simulink model "lab1_extended_estimator"  (R2024b)
settings: Solver=ode45  StartTime=0.0  StopTime=sIn.simulation_time
values from neighbouring files (symbols this model uses):
  Ae = [ref_SS.A_r zeros(3,2); plant_SS.B*ref_SS.C_r plant_SS.A]    [lab1_startup_extended_estimator.m]
  Be = [zeros(3,1); plant_SS.B]    [lab1_startup_extended_estimator.m]
  Ce = [zeros(1,3) plant_SS.C]    [lab1_startup_extended_estimator.m]
undefined symbols (not defined in the file or in its folder): degs2rpm, drv, feedback, filt, gbox, mld, mot, rads2rpm, ref_SS, rpm2rads, sens, sIn, specs
libraries: simulink_extras x2
settings Model: Creator=bmm1  LastModifiedBy=Nihal
settings SolverCC: ZeroCrossAlgorithm=Adaptive
settings DebuggingCC: IgnoredZcDiagnostic=none
settings RTWCC: GPUComputeCapability=3.5

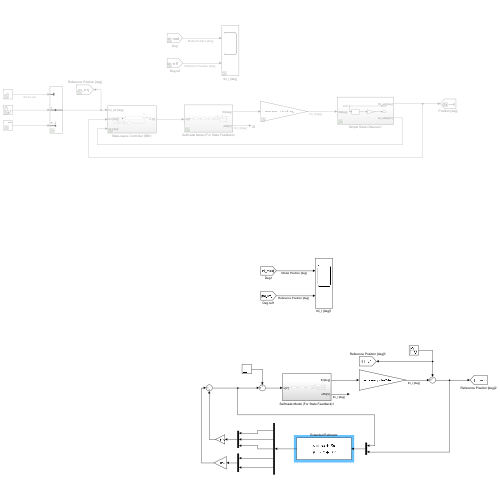
[thumbnail: Simulink's stored preview of the top-level diagram]
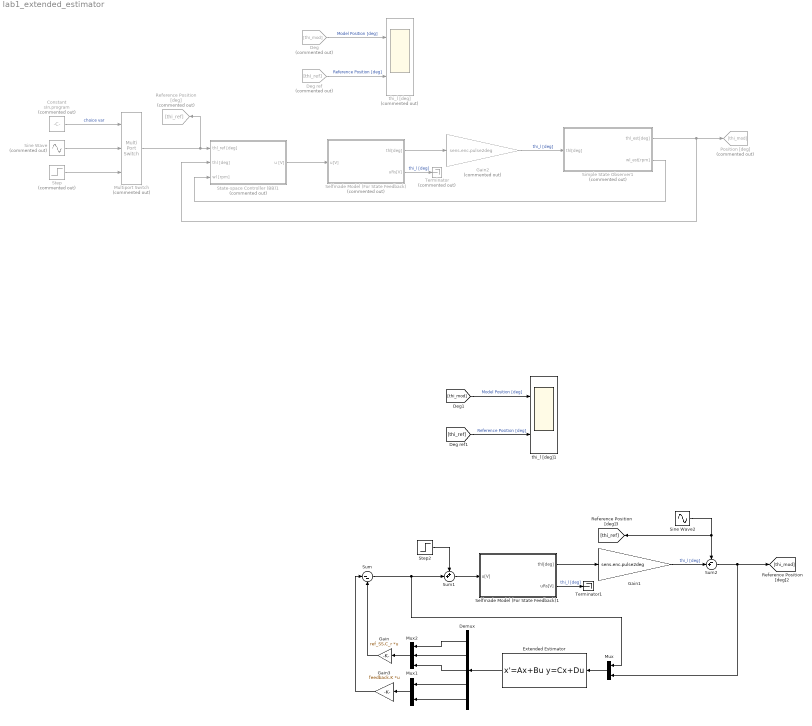
== system lab1_extended_estimator ==
  Constant : Constant  Commented=on  Value=sIn.program
  Deg : From  Commented=on  GotoTag=thi_mod
  Deg ref : From  Commented=on  GotoTag=thi_ref
  Demux : Demux  Outputs=5
  Extended Estimator : StateSpace  A=Ae - feedback.L*Ce  B=[Be, feedback.L]  C=eye(5,5)  D=zeros(5,2)  InitialCondition=0
  Gain : Gain  Gain=ref_SS.C_r  Multiplication=Matrix(K*u)
  Gain1 : Gain  Gain=sens.enc.pulse2deg
  Gain2 : Gain  Commented=on  Gain=sens.enc.pulse2deg
  Gain3 : Gain  Gain=feedback.K  Multiplication=Matrix(K*u)
  Multiport Switch : MultiPortSwitch  Commented=on  Inputs=2  SaturateOnIntegerOverflow=off  InputSameDT=off
  Mux : Mux  Inputs=2
  Mux1 : Mux  Inputs=2
  Mux2 : Mux  Inputs=3
  Position [deg] : Goto  Commented=on  GotoTag=thi_mod
  Reference Position [deg] : Goto  Commented=on  GotoTag=thi_ref
  Selfmade Model (For State Feedback) : Subsystem  Commented=on
  Selfmade Model (For State Feedback)1 : Subsystem
  Simple State Observer1 : Subsystem  Commented=on
  Sine Wave : Sin  Commented=on  Amplitude=specs.Amp  Frequency=specs.Freq  SampleTime=0
  Sine Wave2 : Sin  Amplitude=specs.Amp  Frequency=specs.Freq  SampleTime=0
  State-space Controller (BB)1 : Subsystem  Commented=on
  Step : Step  Commented=on  After=40  SampleTime=0
  Step2 : Step  After=40  SampleTime=0
  Sum : Sum  Inputs=|--
  Sum1 : Sum  Inputs=++|
  Sum2 : Sum  Inputs=-+|
  Terminator : Terminator  Commented=on
  Terminator1 : Terminator
  thi_l [deg] : Scope  Commented=on  NumInputPorts=2
  thi_l [deg]1 : Scope  NumInputPorts=2
  wires:
  Selfmade Model (For State Feedback)/1(thl[deg]) -> Gain2/1
  Deg/1 -> thi_l [deg]/1  "Model Position [deg]"
  Deg ref/1 -> thi_l [deg]/2  "Reference Position [deg]"
  State-space Controller (BB)1/1(u [V]) -> Selfmade Model (For State Feedback)/1(u[V])
  Selfmade Model (For State Feedback)/2(uRs[V]) -> Terminator/1  "thi_l [deg]"
  Gain2/1 -> Simple State Observer1/1(thl[deg])  "thi_l [deg]"
  Simple State Observer1/1(thl_est[deg]) -> Position [deg]/1, State-space Controller (BB)1/2(thl [deg])
  Simple State Observer1/2(wl_est[rpm]) -> State-space Controller (BB)1/3(wl [rpm])
  Sine Wave/1 -> Multiport Switch/2
  Multiport Switch/1 -> Reference Position [deg]/1, State-space Controller (BB)1/1(thl_ref [deg])
  Step/1 -> Multiport Switch/3
  Constant/1 -> Multiport Switch/1  "choice var"
  Selfmade Model (For State Feedback)1/2(uRs[V]) -> Terminator1/1  "thi_l [deg]"
  Sum/1 -> Sum1/2, Mux/1
  [thi_ref] -> thi_l [deg]1/2  "Reference Position [deg]"
  Selfmade Model (For State Feedback)1/1(thl[deg]) -> Gain1/1
  [thi_mod] -> thi_l [deg]1/1  "Model Position [deg]"
  Mux/1 -> Extended Estimator/1
  Extended Estimator/1 -> Demux/1
  Mux1/1 -> Gain3/1
  Demux/4 -> Mux1/1
  Demux/5 -> Mux1/2
  Demux/1 -> Mux2/1
  Demux/2 -> Mux2/2
  Demux/3 -> Mux2/3
  Mux2/1 -> Gain/1
  Gain/1 -> Sum/2
  Gain3/1 -> Sum/1
  Sum1/1 -> Selfmade Model (For State Feedback)1/1(u[V])
  Step2/1 -> Sum1/1
  Gain1/1 -> Sum2/2  "thi_l [deg]"
  Sine Wave2/1 -> Sum2/1, [thi_ref]
  Sum2/1 -> Mux/2, [thi_mod]

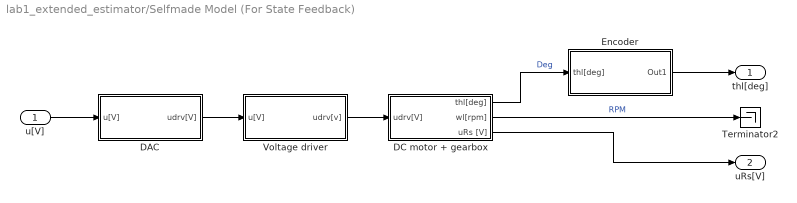
== system lab1_extended_estimator/Selfmade Model (For State Feedback) ==
  u[V] : Inport
  DAC : Subsystem
  DC motor + gearbox : Subsystem
  Encoder : Subsystem
  Terminator2 : Terminator
  Voltage driver : Subsystem
  thl[deg] : Outport
  uRs[V] : Outport  Port=2
  wires:
  DC motor + gearbox/1(thl[deg]) -> Encoder/1(thl[deg])  "Deg"
  u[V]/1 -> DAC/1(u[V])
  DC motor + gearbox/2(wl[rpm]) -> Terminator2/1  "RPM"
  DAC/1(udrv[V]) -> Voltage driver/1(u[V])
  Voltage driver/1(udrv[v]) -> DC motor + gearbox/1(udrv[V])
  Encoder/1(Out1) -> thl[deg]/1
  DC motor + gearbox/3(uRs [V]) -> uRs[V]/1

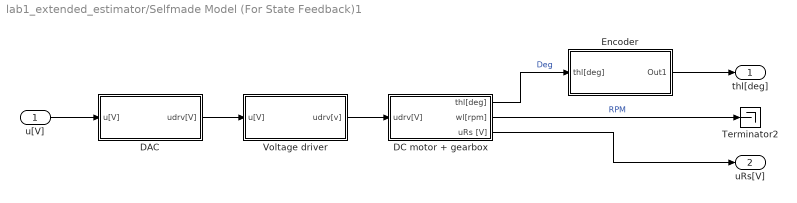
== system lab1_extended_estimator/Selfmade Model (For State Feedback)1 ==
  u[V] : Inport
  DAC : Subsystem
  DC motor + gearbox : Subsystem
  Encoder : Subsystem
  Terminator2 : Terminator
  Voltage driver : Subsystem
  thl[deg] : Outport
  uRs[V] : Outport  Port=2
  wires:
  DC motor + gearbox/1(thl[deg]) -> Encoder/1(thl[deg])  "Deg"
  u[V]/1 -> DAC/1(u[V])
  DC motor + gearbox/2(wl[rpm]) -> Terminator2/1  "RPM"
  DAC/1(udrv[V]) -> Voltage driver/1(u[V])
  Voltage driver/1(udrv[v]) -> DC motor + gearbox/1(udrv[V])
  Encoder/1(Out1) -> thl[deg]/1
  DC motor + gearbox/3(uRs [V]) -> uRs[V]/1

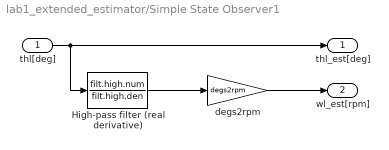
== system lab1_extended_estimator/Simple State Observer1 ==
  thl[deg] : Inport
  High-pass filter (real derivative) : TransferFcn  Numerator=filt.high.num  Denominator=filt.high.den
  degs2rpm : Gain  Gain=degs2rpm
  thl_est[deg] : Outport
  wl_est[rpm] : Outport  Port=2
  wires:
  thl[deg]/1 -> High-pass filter (real derivative)/1, thl_est[deg]/1
  High-pass filter (real derivative)/1 -> degs2rpm/1
  degs2rpm/1 -> wl_est[rpm]/1

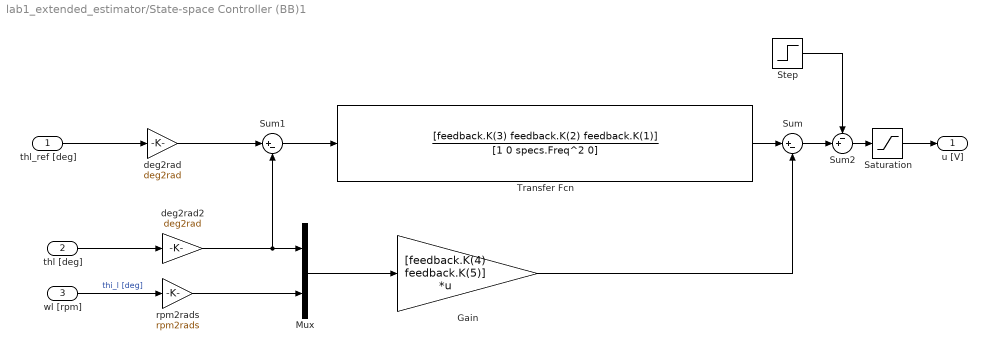
== system lab1_extended_estimator/State-space Controller (BB)1 ==
  thl_ref [deg] : Inport
  thl [deg] : Inport  Port=2
  wl [rpm] : Inport  Port=3
  Gain : Gain  Gain=[feedback.K(4) feedback.K(5)]  Multiplication=Matrix(K*u)
  Mux : Mux  Inputs=2
  Saturation : Saturate  UpperLimit=10  LowerLimit=-10
  Step : Step  After=40  SampleTime=0
  Sum : Sum  Inputs=|+-
  Sum1 : Sum  Inputs=|+-
  Sum2 : Sum  Inputs=-+|
  Transfer Fcn : TransferFcn  Numerator=[feedback.K(3) feedback.K(2) feedback.K(1)]  Denominator=[1 0 specs.Freq^2 0]
  deg2rad : Gain  Gain=deg2rad
  deg2rad2 : Gain  Gain=deg2rad
  rpm2rads : Gain  Gain=rpm2rads
  u [V] : Outport
  wires:
  thl_ref [deg]/1 -> deg2rad/1
  Transfer Fcn/1 -> Sum/1
  Saturation/1 -> u [V]/1
  thl [deg]/1 -> deg2rad2/1
  deg2rad2/1 -> Mux/1, Sum1/2
  deg2rad/1 -> Sum1/1
  Mux/1 -> Gain/1
  rpm2rads/1 -> Mux/2
  Gain/1 -> Sum/2
  Sum1/1 -> Transfer Fcn/1
  wl [rpm]/1 -> rpm2rads/1  "thi_l [deg]"
  Sum2/1 -> Saturation/1
  Sum/1 -> Sum2/2
  Step/1 -> Sum2/1

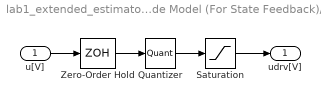
== system lab1_extended_estimator/Selfmade Model (For State Feedback)/DAC ==
  u[V] : Inport
  Quantizer : Quantizer  QuantizationInterval=daq.dac.q
  Saturation : Saturate  UpperLimit=10  LowerLimit=-10
  Zero-Order Hold : ZeroOrderHold  SampleTime=1e-3
  udrv[V] : Outport
  wires:
  Zero-Order Hold/1 -> Quantizer/1
  u[V]/1 -> Zero-Order Hold/1
  Quantizer/1 -> Saturation/1
  Saturation/1 -> udrv[V]/1

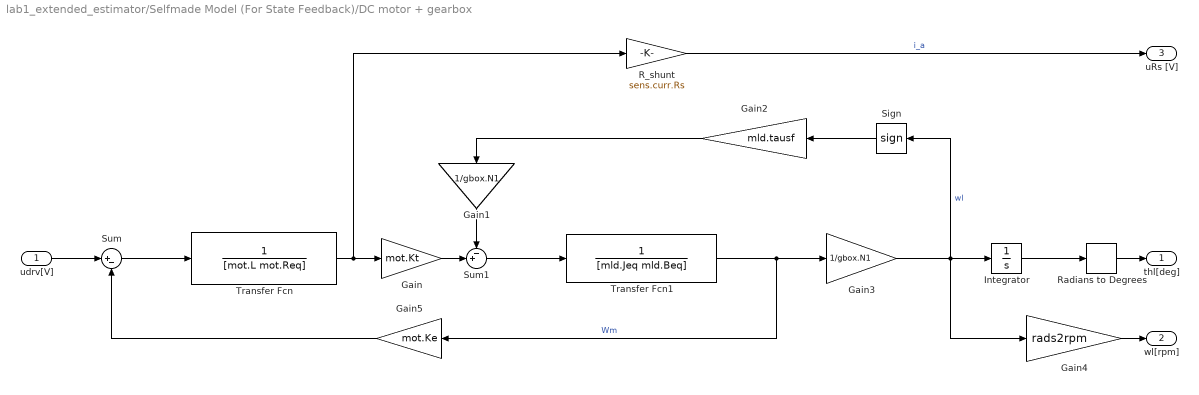
== system lab1_extended_estimator/Selfmade Model (For State Feedback)/DC motor + gearbox ==
  udrv[V] : Inport
  Gain : Gain  Gain=mot.Kt
  Gain1 : Gain  Gain=1/gbox.N1
  Gain2 : Gain  Gain=mld.tausf
  Gain3 : Gain  Gain=1/gbox.N1
  Gain4 : Gain  Gain=rads2rpm
  Gain5 : Gain  Gain=mot.Ke
  Integrator : Integrator
  R_shunt : Gain  Gain=sens.curr.Rs
  Radians to Degrees : simulink_extras/Transformations/Radians to Degrees
  Sign : Signum  ZeroCross=off
  Sum : Sum  Inputs=|+-
  Sum1 : Sum  Inputs=-+|
  Transfer Fcn : TransferFcn  Denominator=[mot.L mot.Req]
  Transfer Fcn1 : TransferFcn  Denominator=[mld.Jeq mld.Beq]
  thl[deg] : Outport
  wl[rpm] : Outport  Port=2
  uRs [V] : Outport  Port=3
  wires:
  udrv[V]/1 -> Sum/1
  Sum/1 -> Transfer Fcn/1
  Transfer Fcn/1 -> R_shunt/1, Gain/1
  Gain1/1 -> Sum1/1
  Gain2/1 -> Gain1/1
  Sign/1 -> Gain2/1
  Transfer Fcn1/1 -> Gain5/1, Gain3/1  "Wm"
  Gain3/1 -> Gain4/1, Sign/1, Integrator/1  "wl"
  Integrator/1 -> Radians to Degrees/1
  Radians to Degrees/1 -> thl[deg]/1
  Gain4/1 -> wl[rpm]/1
  Sum1/1 -> Transfer Fcn1/1
  Gain/1 -> Sum1/2
  Gain5/1 -> Sum/2
  R_shunt/1 -> uRs [V]/1  "i_a"

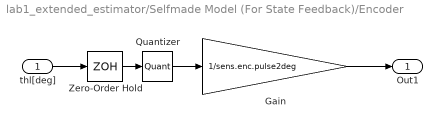
== system lab1_extended_estimator/Selfmade Model (For State Feedback)/Encoder ==
  thl[deg] : Inport
  Gain : Gain  Gain=1/sens.enc.pulse2deg
  Quantizer : Quantizer  QuantizationInterval=sens.enc.pulse2deg
  Zero-Order Hold : ZeroOrderHold  SampleTime=1e-3
  Out1 : Outport
  wires:
  thl[deg]/1 -> Zero-Order Hold/1
  Gain/1 -> Out1/1
  Quantizer/1 -> Gain/1
  Zero-Order Hold/1 -> Quantizer/1

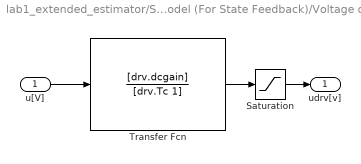
== system lab1_extended_estimator/Selfmade Model (For State Feedback)/Voltage driver ==
  u[V] : Inport
  Saturation : Saturate  UpperLimit=12  LowerLimit=-12
  Transfer Fcn : TransferFcn  Numerator=[drv.dcgain]  Denominator=[drv.Tc 1]
  udrv[v] : Outport
  wires:
  u[V]/1 -> Transfer Fcn/1
  Transfer Fcn/1 -> Saturation/1
  Saturation/1 -> udrv[v]/1

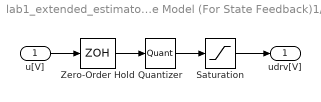
== system lab1_extended_estimator/Selfmade Model (For State Feedback)1/DAC ==
  u[V] : Inport
  Quantizer : Quantizer  QuantizationInterval=daq.dac.q
  Saturation : Saturate  UpperLimit=10  LowerLimit=-10
  Zero-Order Hold : ZeroOrderHold  SampleTime=1e-3
  udrv[V] : Outport
  wires:
  Zero-Order Hold/1 -> Quantizer/1
  u[V]/1 -> Zero-Order Hold/1
  Quantizer/1 -> Saturation/1
  Saturation/1 -> udrv[V]/1

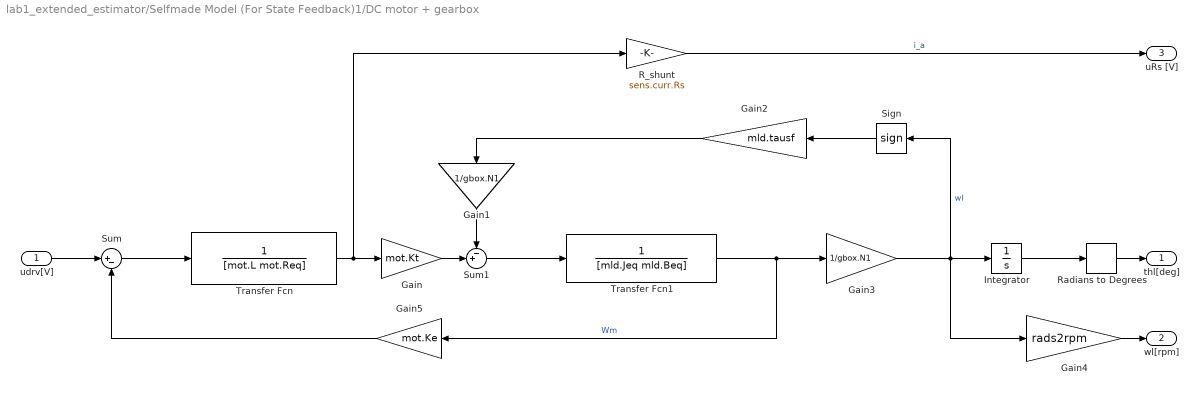
== system lab1_extended_estimator/Selfmade Model (For State Feedback)1/DC motor + gearbox ==
  udrv[V] : Inport
  Gain : Gain  Gain=mot.Kt
  Gain1 : Gain  Gain=1/gbox.N1
  Gain2 : Gain  Gain=mld.tausf
  Gain3 : Gain  Gain=1/gbox.N1
  Gain4 : Gain  Gain=rads2rpm
  Gain5 : Gain  Gain=mot.Ke
  Integrator : Integrator
  R_shunt : Gain  Gain=sens.curr.Rs
  Radians to Degrees : simulink_extras/Transformations/Radians to Degrees
  Sign : Signum  ZeroCross=off
  Sum : Sum  Inputs=|+-
  Sum1 : Sum  Inputs=-+|
  Transfer Fcn : TransferFcn  Denominator=[mot.L mot.Req]
  Transfer Fcn1 : TransferFcn  Denominator=[mld.Jeq mld.Beq]
  thl[deg] : Outport
  wl[rpm] : Outport  Port=2
  uRs [V] : Outport  Port=3
  wires:
  udrv[V]/1 -> Sum/1
  Sum/1 -> Transfer Fcn/1
  Transfer Fcn/1 -> R_shunt/1, Gain/1
  Gain1/1 -> Sum1/1
  Gain2/1 -> Gain1/1
  Sign/1 -> Gain2/1
  Transfer Fcn1/1 -> Gain5/1, Gain3/1  "Wm"
  Gain3/1 -> Gain4/1, Sign/1, Integrator/1  "wl"
  Integrator/1 -> Radians to Degrees/1
  Radians to Degrees/1 -> thl[deg]/1
  Gain4/1 -> wl[rpm]/1
  Sum1/1 -> Transfer Fcn1/1
  Gain/1 -> Sum1/2
  Gain5/1 -> Sum/2
  R_shunt/1 -> uRs [V]/1  "i_a"

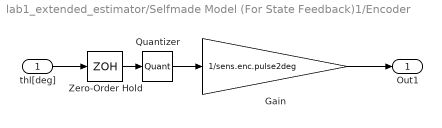
== system lab1_extended_estimator/Selfmade Model (For State Feedback)1/Encoder ==
  thl[deg] : Inport
  Gain : Gain  Gain=1/sens.enc.pulse2deg
  Quantizer : Quantizer  QuantizationInterval=sens.enc.pulse2deg
  Zero-Order Hold : ZeroOrderHold  SampleTime=1e-3
  Out1 : Outport
  wires:
  thl[deg]/1 -> Zero-Order Hold/1
  Gain/1 -> Out1/1
  Quantizer/1 -> Gain/1
  Zero-Order Hold/1 -> Quantizer/1

== system lab1_extended_estimator/Selfmade Model (For State Feedback)1/Voltage driver ==
  u[V] : Inport
  Saturation : Saturate  UpperLimit=12  LowerLimit=-12
  Transfer Fcn : TransferFcn  Numerator=[drv.dcgain]  Denominator=[drv.Tc 1]
  udrv[v] : Outport
  wires:
  u[V]/1 -> Transfer Fcn/1
  Transfer Fcn/1 -> Saturation/1
  Saturation/1 -> udrv[v]/1
